simulink model "SensorEx_Client_Model"  (Simulink 7.6)
settings: Solver=FixedStepDiscrete  StartTime=0.0  StopTime=60  FixedStep=0.1  RelTol=1e-3
libraries: SensorEx_Lib x3, vipsnks x1
settings Model: Creator=Tarex  LastModifiedBy=Tarex
settings DataIOCC: SaveOutput=off  SignalLogging=off  DSMLogging=off  SaveTime=off
settings DebuggingCC: InheritedTsInSrcMsg=none

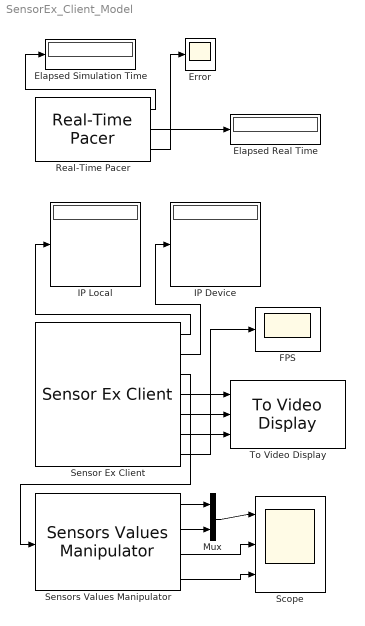
== system SensorEx_Client_Model ==
  Elapsed Real Time : Display
      settings: Decimation=2
  Elapsed Simulation Time : Display
      settings: Decimation=2
  Error : Scope
      settings: YMin=-0.08  YMax=-0.01
  FPS : Scope
      settings: TimeRange=60  YMin=0  YMax=25  SaveName=ScopeData2  SampleInput=on
  IP Device : Display
      settings: Decimation=2
  IP Local : Display
      settings: Decimation=2
  Mux : Mux  Inputs=2
  Real-Time Pacer : SensorEx_Lib/Real-Time Pacer  SystemSampleTime=-1
  Scope : Scope  NumInputPorts=3
      settings: TimeRange=60  YMin=0~-5~-110  YMax=70~11~50  SampleInput=on
  Sensor Ex Client : SensorEx_Lib/Sensor Ex Client  deviceNumber=2  imgSize=[320 240]
  Sensors Values Manipulator : SensorEx_Lib/Sensors Values Manipulator  SystemSampleTime=-1  outType=Standard  outStampT=on
  To Video Display : vipsnks/To Video Display  DialogControllerArgs=DataTag0  inputType=Obsolete  imagePorts=Separate color signals  OutputDevice=On-screen video monitor  fullScreen=off  videoWindowX=208  videoWindowY=4  saveWindowSize=off  videoWindowWidth=240  videoWindowHeight=320  dataOrg=Column-major  openAtMdlStart=on  isWindowOpen=on
  wires:
  Real-Time Pacer/1 -> Elapsed Simulation Time/1
  Real-Time Pacer/2 -> Elapsed Real Time/1
  Real-Time Pacer/3 -> Error/1
  Sensor Ex Client/3 -> Sensors Values Manipulator/1
  Sensor Ex Client/4 -> To Video Display/1
  Sensor Ex Client/5 -> To Video Display/2
  Sensor Ex Client/6 -> To Video Display/3
  Sensor Ex Client/1 -> IP Local/1
  Sensor Ex Client/2 -> IP Device/1
  Sensor Ex Client/7 -> FPS/1
  Sensors Values Manipulator/2 -> Mux/2
  Sensors Values Manipulator/1 -> Mux/1
  Mux/1 -> Scope/1
  Sensors Values Manipulator/4 -> Scope/3
  Sensors Values Manipulator/3 -> Scope/2
